simulink library "thc"  (R2021b)
settings: Solver=VariableStepAuto  StartTime=0.0  StopTime=10.0  RelTol=1e-3
undefined symbols (not defined in the file or in its folder): ATHC_APTCQA_X_C, ATHC_APTCQB_X_C, ATHC_dAy_X_C, ATHC_Qeq_X_kmh, ATHC_VbaseC_X_C, ATHC_VbaseC_Y_W, ATHC_VbaseD_X_C, ATHC_VbaseH_X_C, FALSE, KTHC_ACMaxMinT_sec, KTHC_aDeice_K, KTHC_AGSDefLv_K, KTHC_AGSLv1_K, KTHC_AGSLv2_K, KTHC_AGSLv3_K, KTHC_AGSLv4_K, KTHC_AGSLv5_K, KTHC_AirIntUpdateT_sec, KTHC_APTCOneZoneMax_W, KTHC_APTCPeriod_cnt, KTHC_APTCPWMEN_flg, KTHC_APTCQMaxC_W, KTHC_APTCQminC_W, KTHC_APTCQminD_W, KTHC_APTCQminRe1_W, KTHC_APTCQminRe_W, KTHC_APTCQoffT_cnt, KTHC_APTCQonT_cnt, KTHC_APTCRiLeMaxDff_W, KTHC_APTCRiLeMinDff_W, KTHC_BatInTempDef_C, KTHC_bDeice_K, KTHC_CompMaxDeice_rpm, KTHC_CompMinDeice_rpm, KTHC_CompSotxvOp_K, KTHC_CompSotxvOpLow_rpm, KTHC_CompSpdmax_rpm, KTHC_CompSpdmaxBC1_rpm, KTHC_CompSpdmaxBC_rpm, KTHC_CompSpdmid1_rpm, KTHC_CompSpdmid2_rpm, KTHC_CompSpdmid3_rpm, KTHC_CompSpdmid_rpm, KTHC_CompSpdmin_rpm, KTHC_DAPTCQ1_W, KTHC_DAPTCQ2_W, KTHC_DAPTCQ3_W, KTHC_DcChSetTemp_C, KTHC_DehumidityEN_flg, KTHC_DeiceCycTime_K, KTHC_DriveLevelWPTCBAH1_W, KTHC_DriveLevelWPTCBAH2_W, KTHC_DriveLevelWPTCBAH3_W, KTHC_DriveLevelWPTCBAH4_W, KTHC_DriveT1MinBAH_C, KTHC_DriveT2MaxBAH_C, KTHC_DriveT2MinBAH_C, KTHC_DriveT3MaxBAH_C, KTHC_DriveT3MinBAH_C, KTHC_DriveT4MaxBAH_C ... (+377)
libraries: simulink x145
(part 3 of 10)

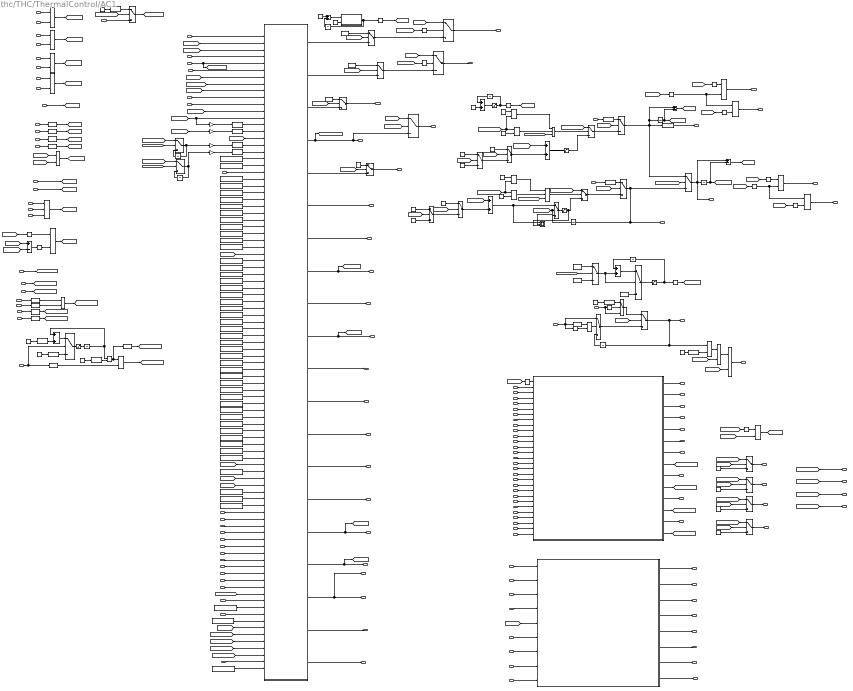
== system thc/THC/ThermalControl/AC1 ==
  VINP_FCPFrEvtBtnACMaxReq_flg : Inport
  VINP_FCPFrEvtBtnACReq_flg : Inport  Port=2
  VINP_FCPFrEvtBtnAutoReq_flg : Inport  Port=3
  VINP_FCPFrEvtBtnSyncReq_flg : Inport  Port=4
  VINP_Tamb_C : Inport  Port=5
  VINP_Tincar_C : Inport  Port=6
  VINP_sigAirIntenZon1Req_enum : Inport  Port=7
  VINP_sigRecircReq_flg : Inport  Port=8
  VINP_sigFaceReq_flg : Inport  Port=9
  VINP_sigFootReq_flg : Inport  Port=10
  VINP_sigFrostReq_flg : Inport  Port=11
  VINP_sigSetTempZon1Req_C : Inport  Port=12
  VINP_CANMsgValidIVI2_flg : Inport  Port=13
  VINP_sigSetTempZon2Req_C : Inport  Port=14
  VTHC_FDBlowerCmd_pct : Inport  Port=15
  PwrSta : Inport  Port=16
  OFF_AC_MODE : Inport  Port=17
  CabinMode : Inport  Port=18
  T_Foot_L : Inport  Port=19
  T_Foot_R : Inport  Port=20
  T_Foot_Rr : Inport  Port=21
  EEP_ACModeMem : Inport  Port=22
  EEP_Face : Inport  Port=23
  EEP_Foot : Inport  Port=24
  EEP_Frost : Inport  Port=25
  EEP_FaceM : Inport  Port=26
  EEP_FootM : Inport  Port=27
  EEP_CCUSyncSts : Inport  Port=28
  EEP_ACForceOFF : Inport  Port=29
  EEP_sigRecircSt : Inport  Port=30
  EEP_RecAutoFlg : Inport  Port=31
  EEP_AirIntenZone1M : Inport  Port=32
  EEP_fdefog : Inport  Port=33
  EEP_sigSetTempZon1Req : Inport  Port=34
  EEP_sigSetTempZon2StM : Inport  Port=35
  VINP_RemoteAutoReq_flg : Inport  Port=36
  ACSubMode : Inport  Port=37
  VINP_HMIACBtnCmd_flg : Inport  Port=38
  VINP_HMIACAutoBtnCmd_flg : Inport  Port=39
  VINP_HMIACRecycleBtnCmd_flg : Inport  Port=40
  VINP_HMIACFrDefogBtnCmd_flg : Inport  Port=41
  VINP_HMIZ1SetTPCmd_flg : Inport  Port=42
  VINP_HMIZ1SetTMCmd_flg : Inport  Port=43
  VINP_HMIZ2SetTPCmd_flg : Inport  Port=44
  VINP_HMIZ2SetTMCmd_flg : Inport  Port=45
  VINP_HMIACWindDirPCmd_flg : Inport  Port=46
  VINP_HMIACWindDirMCmd_flg : Inport  Port=47
  VINP_HMIACAirIntPCmd_flg : Inport  Port=48
  VINP_HMIACAirIntDirMCmd_flg : Inport  Port=49
  VINP_IVIAirIntZ3Cmd_enum : Inport  Port=50
  EEP_FDCTHCAirIntZ3Sta : Inport  Port=51
  VINP_IVIDrBlowerModeSta_enum : Inport  Port=52
  VINP_IVIPsBlowerModeSta_enum : Inport  Port=53
  VINP_IVIDrBlowerZSta_enum : Inport  Port=54
  VINP_IVICLBlowerZSta_enum : Inport  Port=55
  VINP_IVIPsBlowerZSta_enum : Inport  Port=56
  VINP_IVICRBlowerZSta_enum : Inport  Port=57
  VINP_IVIDrBlowerYSta_enum : Inport  Port=58
  VINP_IVICLBlowerYSta_enum : Inport  Port=59
  VINP_IVIPsBlowerYSta_enum : Inport  Port=60
  VINP_IVICRBlowerYSta_enum : Inport  Port=61
  VINP_ZFRTHCDrEVentActYSta_enum : Inport  Port=62
  VINP_ZFRTHCCLEVentActYSta_enum : Inport  Port=63
  VINP_ZFRTHCPsEVentActYSta_enum : Inport  Port=64
  VINP_ZFRTHCCREVentActYSta_enum : Inport  Port=65
  VINP_FDCTHCDrEVentModeStaM_enum : Inport  Port=66
  VINP_FDCTHCPsEVentModeStaM_enum : Inport  Port=67
  VINP_FDCTHCDrEVentZStaM_enum : Inport  Port=68
  VINP_FDCTHCCLEVentZStaM_enum : Inport  Port=69
  VINP_FDCTHCPsEVentZStaM_enum : Inport  Port=70
  VINP_FDCTHCCREVentZStaM_enum : Inport  Port=71
  EEP_DrVentENM : Inport  Port=72
  VINP_FDCTHCDrEVentYStaM_enum : Inport  Port=73
  EEP_CLVentENM : Inport  Port=74
  VINP_FDCTHCCLEVentYStaM_enum : Inport  Port=75
  EEP_PsVentENM : Inport  Port=76
  VINP_FDCTHCPsEVentYStaM_enum : Inport  Port=77
  EEP_CRVentENM : Inport  Port=78
  VINP_FDCTHCCREVentYStaM_enum : Inport  Port=79
  VINP_IVIsigScreenReq_Sta : Inport  Port=80
  VINP_IVIFGSAirIntCmd_enum : Inport  Port=81
  FGSAirIntStaM : Inport  Port=82
  VINP_IVIFGSChCmd_enum : Inport  Port=83
  FGSChStaM : Inport  Port=84
  VINP_IVIIONSWCmd_flg : Inport  Port=85
  "IONSWStaM " : Inport  Port=86
  VINP_FGSMotorInitSta_enum : Inport  Port=87
  VINP_FGSAirIntSta_enum : Inport  Port=88
  VINP_IVIZon1WindDirSWReqSta_flg : Inport  Port=89
  Add{,1..2,4..6} (6 alike) : Sum
  Add3 : Sum  Inputs=+-
  Add7 : Sum  Inputs=+-
  Add8 : Sum  Inputs=+-
  Chart : Stateflow chart  TreatAsAtomicUnit=on
      settings: PortSchema="{\"entries\":[{\"content\":{\"sides\":[{\"content\":{\"connectorIds\":[\"In1\",\"In2\",\"In3\",\"In4\",\"In5\",\"In6\",\"In7\",\"In8\",\"In9\",\"In10\",\"In11\",\"In12\",\"In13\",\"In14\",\"In15\",\"In16\",\"In18\",\"In17\",\"In19\",\"In20\",\"In21\",\"In22\",\"In23\",\"In24\",\"In25\",\"In26\",\"In27\",\"In28\",\"In29\",\"In30\",\"In31\",\"In32\",\"In33\",\"In34\",\"In35\",\"In36\",\"In37\",\"In38\",\"In39\",\"In40\",\"In41\",\"In42\",\"In43\",\"In44\",\"In45\",\"In46\",\"In47\",\"In48\",\"In49\",\"In50\",\"In51\",\"In52\",\"In53\",\"In54\",\"In55\",\"In56\",\"In57\",\"In58\",\"In59\",\"In60\",\"In61\",\"In62\",\"In63\",\"In64\",\"In65\",\"In66\",\"In67\",\"In68\",\"In69\",\"In70\",\"In71\",\"In72\",\"In73\",\"In74\",\"In75\",\"In76\",\"In77\",\"In78\",\"In79\",\"In80\",\"In81\",\"In82\",\"In83\",\"In84\",\"In85\",\"In86\",\"In87\",\"In88\",\"In89\",\"In90\",\"In91\",\"In92\",\"In93\",\"In94\"]},\"type\":\"ConnectorPlacement.EquallySpacedRectSide\",\"uuid\":\"5820fc40-35f0-4b43-a348-a95be02a5108\"},{\"content\":{\"connectorIds\":[\"Out1\",\"Out6\",\"Out2\",\"Out3\",\"Out4\",\"Out5\",\"Out7\",\"Out8\",\"Out9\",\"Out10\",\"Out11\",\"Out12\",\"Out13\",\"Out14\",\"Out15\",\"Out16\",\"Out17\",\"Out18\",\"Out19\",\"Out20\"],\"side\":\"RIGHT\"},\"type\":\"ConnectorPlacement.EquallySpacedRectSide\",\"uuid\":\"36d6613c-bf09-4a00-b7cd-6c94d14300cf\"},{\"content\":{\"connectorIds\":[],\"side\":\"TOP\"},\"type\":\"ConnectorPlacement.EquallySpacedRectSide\",\"uuid\":\"1ae2c247-46e8-45cc-9ea1-ac445f4d9fda\"}]},\"type\":\"ConnectorPlacement.EquallySpacedConnector\",\"uuid\":\"a8684177-dc23-416a-a392-32f98192c4b4\"}],\"packageUris\":[\"http://schema.mathworks.com/mf0/Connector/R2020b\"],\"version\":\"1.0\"}"
  Compare To Constant : simulink/Logic and Bit Operations/Compare To Constant  relop=<  const=5  OutDataTypeStr=boolean
  Compare To Constant1 : simulink/Logic and Bit Operations/Compare To Constant  relop=>=  const=1  OutDataTypeStr=boolean
  Compare To Constant10 : simulink/Logic and Bit Operations/Compare To Constant  relop=>  const=0  OutDataTypeStr=boolean
  Compare To Constant11 : simulink/Logic and Bit Operations/Compare To Constant  relop=<  const=0  OutDataTypeStr=boolean
  Compare To Constant12 : simulink/Logic and Bit Operations/Compare To Constant  relop=>  const=0  OutDataTypeStr=boolean
  Compare To Constant13 : simulink/Logic and Bit Operations/Compare To Constant  relop=<  const=0  OutDataTypeStr=boolean
  Compare To Constant2 : simulink/Logic and Bit Operations/Compare To Constant  relop=>=  const=100  OutDataTypeStr=boolean
  Compare To Constant3 : simulink/Logic and Bit Operations/Compare To Constant  relop===  const=3.0  OutDataTypeStr=boolean
  Compare To Constant4 : simulink/Logic and Bit Operations/Compare To Constant  relop=<  const=0  OutDataTypeStr=boolean
  Compare To Constant5 : simulink/Logic and Bit Operations/Compare To Constant  relop=<  const=3.0  OutDataTypeStr=boolean
  Compare To Constant6 : simulink/Logic and Bit Operations/Compare To Constant  relop===  const=2  OutDataTypeStr=boolean
  Compare To Constant7 : simulink/Logic and Bit Operations/Compare To Constant  relop===  const=1  OutDataTypeStr=boolean
  Compare To Constant8 : simulink/Logic and Bit Operations/Compare To Constant  relop===  const=0  OutDataTypeStr=boolean
  Compare To Constant9 : simulink/Logic and Bit Operations/Compare To Constant  relop=>  const=0  OutDataTypeStr=boolean
  Constant{,8,55,68,70..71} (6 alike) : Constant
  Constant1 : Constant  Value=10
  Constant10 : Constant  Value=KTHC_T2Mmaxamb_C
  Constant11 : Constant  Value=KTHC_T3Mmaxamb_C
  Constant12 : Constant  Value=KTHC_T4Mmaxamb_C
  Constant13 : Constant  Value=KTHC_T3Mminamb_C
  Constant14 : Constant  Value=KTHC_T4Mminamb_C
  Constant15 : Constant  Value=KTHC_T5Mminamb_C
  Constant16 : Constant  Value=KTHC_RecyHold_min
  Constant17 : Constant  Value=KTHC_RecyChange_min
  Constant18 : Constant  Value=KTHC_Tmidlevel_C
  Constant19 : Constant  Value=KTHC_Thilevel1_C
  Constant2 : Constant  Value=FALSE
  Constant20 : Constant  Value=KTHC_Thilevel2_C
  Constant21 : Constant  Value=KTHC_WDZ1Face_flg
  Constant22 : Constant  Value=KTHC_WDZ1Foot_flg
  Constant23 : Constant  Value=KTHC_WDZ1Frost_flg
  Constant24 : Constant  Value=KTHC_WDZ2Face_flg
  Constant25 : Constant  Value=KTHC_WDZ2Foot_flg
  Constant26 : Constant  Value=KTHC_WDZ2Frost_flg
  Constant27 : Constant  Value=KTHC_WDZ3Face_flg
  Constant28 : Constant  Value=KTHC_WDZ3Foot_flg
  Constant29 : Constant  Value=KTHC_WDZ3Frost_flg
  Constant3 : Constant  Value=FALSE
  Constant30 : Constant  Value=KTHC_WDZ4Face_flg
  Constant31 : Constant  Value=KTHC_WDZ4Foot_flg
  Constant32 : Constant  Value=KTHC_WDZ4Frost_flg
  Constant33 : Constant  Value=KTHC_WDZ5Face_flg
  Constant34 : Constant  Value=KTHC_WDZ5Foot_flg
  Constant35 : Constant  Value=KTHC_WDZ5Frost_flg
  Constant36 : Constant  Value=KTHC_WDZ6Face_flg
  Constant37 : Constant  Value=KTHC_WDZ6Foot_flg
  Constant38 : Constant  Value=KTHC_WDZ6Frost_flg
  Constant39 : Constant  Value=KTHC_WDZ7Face_flg
  Constant4 : Constant  Value=ZERO_INT
  Constant40 : Constant  Value=KTHC_WDZ7Foot_flg
  Constant41 : Constant  Value=KTHC_WDZ7Frost_flg
  Constant42 : Constant  Value=KTHC_WDZ8Face_flg
  Constant43 : Constant  Value=KTHC_WDZ8Foot_flg
  Constant44 : Constant  Value=KTHC_WDZ8Frost_flg
  Constant45 : Constant  Value=KTHC_WDZ9Face_flg
  Constant46 : Constant  Value=KTHC_WDZ9Foot_flg
  Constant47 : Constant  Value=KTHC_WDZ9Frost_flg
  Constant48 : Constant  Value=ONE_INT
  Constant49 : Constant  Value=ZERO_INT
  Constant5 : Constant  Value=KTHC_RecyOutterD_enum
  Constant50 : Constant  Value=KTHC_Trecymin_C
  Constant51 : Constant  Value=KTHC_RefreshEN_flg
  Constant52 : Constant  Value=KTHC_FootColdT_C
  Constant53 : Constant  Value=KTHC_FootColdTdelta_C
  Constant54 : Constant  Value=KTHC_ACMaxMinT_sec
  Constant56 : Constant  Value=FALSE
  Constant57 : Constant  Value=KTHC_WDZ10Foot_flg
  Constant58 : Constant  Value=KTHC_WDZ10Frost_flg
  Constant59 : Constant  Value=0.5
  Constant6 : Constant  Value=KTHC_WDZ10Face_flg
  Constant60 : Constant  Value=-0.5
  Constant61 : Constant  Value=0
  Constant62 : Constant  Value=0.5
  Constant63 : Constant  Value=-0.5
  Constant64 : Constant  Value=0
  Constant65 : Constant  Value=32
  Constant66 : Constant  Value=32
  Constant67 : Constant  Value=0
  Constant69 : Constant  Value=11
  Constant7 : Constant  Value=KTHC_WindDirUpdateT_min
  Constant{72..75} (4 alike) : Constant  Value=false
  Constant76 : Constant  Value=4
  Constant77 : Constant  Value=17
  Constant78 : Constant  Value=17
  Constant79 : Constant  Value=KTHC_ScreenUniq_flg
  Constant9 : Constant  Value=KTHC_AirIntUpdateT_sec
  Data Type Conversion : DataTypeConversion  OutDataTypeStr=single
  Data Type Conversion1 : DataTypeConversion  OutDataTypeStr=single
  Data Type Conversion{6..11} (6 alike) : DataTypeConversion  OutDataTypeStr=uint8
  Data Type Conversion12 : DataTypeConversion  OutDataTypeStr=single
  Data Type Conversion{2..5} (4 alike) : DataTypeConversion  OutDataTypeStr=uint16
  Detect Change : simulink/Logic and Bit Operations/Detect Change  vinit=0  OutDataTypeStr=boolean
  Detect Decrease : simulink/Logic and Bit Operations/Detect Decrease  vinit=0.0  OutDataTypeStr=boolean
  Detect Decrease1 : simulink/Logic and Bit Operations/Detect Decrease  vinit=0.0  OutDataTypeStr=boolean
  Detect Increase{,1..7} (8 alike) : simulink/Logic and Bit Operations/Detect Increase  vinit=0.0  OutDataTypeStr=boolean
  EVent : Subsystem
  Gain{,1..3} (4 alike) : Gain  Gain=10
  Logical Operator : Logic  Operator=NXOR  AllPortsSameDT=off  OutDataTypeStr=boolean
  Logical Operator{1..2,4..6,11,20} (7 alike) : Logic  Operator=OR  AllPortsSameDT=off  OutDataTypeStr=boolean
  Logical Operator{3,9..10,12..16} (8 alike) : Logic  AllPortsSameDT=off  OutDataTypeStr=boolean
  Logical Operator17 : Logic  Operator=NOT  AllPortsSameDT=off  OutDataTypeStr=boolean
  Logical Operator18 : Logic  Operator=NOT  AllPortsSameDT=off  OutDataTypeStr=boolean
  Logical Operator19 : Logic  Operator=NOT  AllPortsSameDT=off  OutDataTypeStr=boolean
  Logical Operator7 : Logic  Inputs=3  AllPortsSameDT=off  OutDataTypeStr=boolean
  Logical Operator8 : Logic  Inputs=3  AllPortsSameDT=off  OutDataTypeStr=boolean
  Min : MinMax  Inputs=3
  ModMath2 : Subsystem  mask(Count){}
      mask help: Counter function.
      mask Display:
      | fprintf('ModMath');
      | port_label('output', 1, 'Remainder');
      | port_label('input', 1, 'Dividend');
      | port_label('input', 2, 'Divisor');
  Relational Operator{,1,4..5} (4 alike) : RelationalOperator  Operator=<=  OutDataTypeStr=boolean  RndMeth=Simplest
  Relational Operator2 : RelationalOperator  Operator=<  OutDataTypeStr=boolean  RndMeth=Simplest
  Relational Operator3 : RelationalOperator  Operator=>  OutDataTypeStr=boolean  RndMeth=Simplest
  Saturation : Saturate  UpperLimit=100  LowerLimit=0
  Saturation1 : Saturate  UpperLimit=3  LowerLimit=0
  Saturation2 : Saturate  UpperLimit=32  LowerLimit=17
  Saturation3 : Saturate  UpperLimit=32  LowerLimit=17
  Saturation4 : Saturate  UpperLimit=12  LowerLimit=0
  Scope : Scope  NumInputPorts=3
  Subsystem : Subsystem
  Switch{,1..29} (30 alike) : Switch  Criteria=u2 > Threshold
  Unit Delay{,2,4..10} (9 alike) : UnitDelay  SampleTime=-1  HasFrameUpgradeWarning=on
  Unit Delay1 : UnitDelay  InitialCondition=26  SampleTime=-1  HasFrameUpgradeWarning=on
  VTHC_CCUACLampSts_flg : Outport
  VTHC_CCUAutoLampSts_flg : Outport  Port=2
  VTHC_CCUACMaxLampSts_flg : Outport  Port=3
  VTHC_CCUSyncLampSts_flg : Outport  Port=4
  VTHC_sigAirIntenZon1St_enum : Outport  Port=5
  VTHC_sigWindDirZon1St_enum : Outport  Port=6
  VTHC_sigRecircSt_flg : Outport  Port=7
  VTHC_sigSetTempZon1St_C : Outport  Port=8
  VTHC_sigSetTempZon2St_C : Outport  Port=9
  WaterFillReq : Outport  Port=10
  PET : Outport  Port=11
  FD_RecyAuto_Cmd : Outport  Port=12
  ACModeMem : Outport  Port=13
  Face : Outport  Port=14
  Foot : Outport  Port=15
  Frost : Outport  Port=16
  FaceM : Outport  Port=17
  FootM : Outport  Port=18
  CCUSyncSts : Outport  Port=19
  ACForceOFF : Outport  Port=20
  RecAutoFlg : Outport  Port=21
  AirIntenZone1M : Outport  Port=22
  fdefog : Outport  Port=23
  VTHC_sigSetTempZon2StM_C : Outport  Port=24
  VTHC_sigDfrstSt_flg : Outport  Port=25
  VTHC_FDCTHCAirIntZ3Sta_enum : Outport  Port=26
  RrAPTCEN : Outport  Port=27
  VTHC_FDCTHCDrEVentModeSta_enum : Outport  Port=28
  VTHC_FDCTHCPsEVentModeSta_enum : Outport  Port=29
  VTHC_FDCTHCDrEVentZSta_enum : Outport  Port=30
  VTHC_FDCTHCCLEVentZSta_enum : Outport  Port=31
  VTHC_FDCTHCPsEVentZSta_enum : Outport  Port=32
  VTHC_FDCTHCCREVentZSta_enum : Outport  Port=33
  VTHC_FDCTHCDrEVentYSta_enum : Outport  Port=34
  VTHC_FDCTHCDrVentENSta_flg : Outport  Port=35
  VTHC_FDCTHCCLEVentYSta_enum : Outport  Port=36
  VTHC_FDCTHCCLVentENSta_flg : Outport  Port=37
  VTHC_FDCTHCPsEVentYSta_enum : Outport  Port=38
  VTHC_FDCTHCPsVentENSta_flg : Outport  Port=39
  VTHC_FDCTHCCREVentYSta_enum : Outport  Port=40
  VTHC_FDCTHCCRVentENSta_flg : Outport  Port=41
  VTHC_DrVentEN_flg : Outport  Port=42
  VTHC_CLVentEN_flg : Outport  Port=43
  VTHC_PsVentEN_flg : Outport  Port=44
  VTHC_CRVentEN_flg : Outport  Port=45
  VTHC_Z1TUP_flg : Outport  Port=46
  VTHC_Z1TDN_flg : Outport  Port=47
  VTHC_Z2TUP_flg : Outport  Port=48
  VTHC_Z2TDN_flg : Outport  Port=49
  VTHC_FDCFGSAirIntSta_enum : Outport  Port=50
  VTHC_FDCFGSChSta_enum : Outport  Port=51
  VTHC_FDCFGSAirIntCmd_enum : Outport  Port=52
  VTHC_FDCFGSFuncSta_flg : Outport  Port=53
  VTHC_FDCFGSChCmd_enum : Outport  Port=54
  VTHC_FDCFGSIONSWSta_flg : Outport  Port=55
  VTHC_FDCFGSIONCmd_flg : Outport  Port=56
  VTHC_FDCFGSLearnCmd_enum : Outport  Port=57
  wires:
  Logical Operator16/1 -> VTHC_Z2TDN_flg/1  "VTHC_Z2TDN_flg"
  [Z2TempG] -> Compare To Constant13/1
  Logical Operator15/1 -> VTHC_Z2TUP_flg/1  "VTHC_Z2TUP_flg"
  Compare To Constant13/1 -> Logical Operator16/2
  Switch12/1 -> Unit Delay1/1, VTHC_sigSetTempZon2StM_C/1, Switch/3  "VTHC_sigSetTempZon2StM_C"
  Compare To Constant12/1 -> Logical Operator15/1
  [Z2TempG] -> Compare To Constant12/1
  Add8/1 -> [Z2TempG]
  Logical Operator19/1 -> Logical Operator16/1, Logical Operator15/2
  Logical Operator14/1 -> VTHC_Z1TDN_flg/1  "VTHC_Z1TDN_flg"
  [Z1TempG] -> Compare To Constant11/1
  Unit Delay10/1 -> [sigSetTempZon1St], Add7/2
  Switch11/1 -> Unit Delay10/1, Add7/1, Switch/1, Data Type Conversion12/1  "VTHC_sigSetTempZon1St_C"
  Add7/1 -> [Z1TempG]
  Compare To Constant11/1 -> Logical Operator14/2
  Compare To Constant10/1 -> Logical Operator13/1
  Logical Operator13/1 -> VTHC_Z1TUP_flg/1  "VTHC_Z1TUP_flg"
  Logical Operator17/1 -> Logical Operator14/1, Logical Operator13/2
  [Z1TempG] -> Compare To Constant10/1
  [DrVentEN] -> VTHC_DrVentEN_flg/1
  [CLVentEN] -> VTHC_CLVentEN_flg/1
  [PSVentEN] -> VTHC_PsVentEN_flg/1
  [CRVentEN] -> VTHC_CRVentEN_flg/1
  Data Type Conversion12/1 -> VTHC_sigSetTempZon1St_C/1  "VTHC_sigSetTempZon1St_C"
  VINP_IVIsigScreenReq_Sta/1 -> Chart/93(sigScreenReq)
  Logical Operator12/1 -> [EVACEN]
  [Face] -> Logical Operator12/2
  Compare To Constant9/1 -> Logical Operator12/1
  [VTHC_FDBlowerCmd_pct] -> Compare To Constant9/1
  Constant76/1 -> Data Type Conversion11/1
  Data Type Conversion11/1 -> Switch29/1
  EEP_FDCTHCAirIntZ3Sta/1 -> Compare To Constant8/1, Switch29/3
  Compare To Constant8/1 -> Switch29/2
  EVent/14(VTHC_FDCTHCCRVentEN_flg) -> [CRVentEN]
  [CRVentEN] -> Switch28/1
  [EVACEN] -> Switch28/2
  Constant75/1 -> Switch28/3
  EVent/12(VTHC_FDCTHCPsVentEN_flg) -> [PSVentEN]
  Constant74/1 -> Switch27/3
  [EVACEN] -> Switch27/2
  [PSVentEN] -> Switch27/1
  EVent/10(VTHC_FDCTHCCLVentEN_flg) -> [CLVentEN]
  [CLVentEN] -> Switch26/1
  [EVACEN] -> Switch26/2
  Constant73/1 -> Switch26/3
  Constant72/1 -> Switch25/3
  [EVACEN] -> Switch25/2
  [DrVentEN] -> Switch25/1
  EVent/8(VTHC_FDCTHCDrVentEN_flg) -> [DrVentEN]
  Switch25/1 -> VTHC_FDCTHCDrVentENSta_flg/1
  Switch28/1 -> VTHC_FDCTHCCRVentENSta_flg/1
  EVent/13(VTHC_FDCTHCCREVentYSta_enum) -> VTHC_FDCTHCCREVentYSta_enum/1
  Switch27/1 -> VTHC_FDCTHCPsVentENSta_flg/1
  EVent/11(VTHC_FDCTHCPsEVentYSta_enum) -> VTHC_FDCTHCPsEVentYSta_enum/1
  Switch26/1 -> VTHC_FDCTHCCLVentENSta_flg/1
  EVent/9(VTHC_FDCTHCCLEVentYSta_enum) -> VTHC_FDCTHCCLEVentYSta_enum/1
  EVent/7(VTHC_FDCTHCDrEVentYSta_enum) -> VTHC_FDCTHCDrEVentYSta_enum/1
  EVent/6(VTHC_FDCTHCCREVentZSta_enum) -> VTHC_FDCTHCCREVentZSta_enum/1
  EVent/5(VTHC_FDCTHCPsEVentZSta_enum) -> VTHC_FDCTHCPsEVentZSta_enum/1
  EVent/4(VTHC_FDCTHCCLEVentZSta_enum) -> VTHC_FDCTHCCLEVentZSta_enum/1
  EVent/3(VTHC_FDCTHCDrEVentZSta_enum) -> VTHC_FDCTHCDrEVentZSta_enum/1
  EVent/2(VTHC_FDCTHCPsEVentModeSta_enum) -> VTHC_FDCTHCPsEVentModeSta_enum/1
  EVent/1(VTHC_FDCTHCDrEVentModeSta_enum) -> VTHC_FDCTHCDrEVentModeSta_enum/1
  Logical Operator11/1 -> RrAPTCEN/1
  [Foot] -> Logical Operator11/2
  Logical Operator10/1 -> Logical Operator11/1
  Relational Operator3/1 -> Logical Operator10/1
  [Face] -> Logical Operator10/2
  Data Type Conversion10/1 -> Relational Operator3/2
  Constant71/1 -> Data Type Conversion10/1
  VINP_FDCTHCCREVentYStaM_enum/1 -> EVent/29(VINP_FDCTHCCREVentYStaM_enum)
  EEP_CRVentENM/1 -> EVent/28(VTHC_FDCTHCCRVentENM_flg)
  VINP_FDCTHCPsEVentYStaM_enum/1 -> EVent/26(VINP_FDCTHCPsEVentYStaM_enum)
  EEP_PsVentENM/1 -> EVent/25(VTHC_FDCTHCPsVentENM_flg)
  VINP_FDCTHCCLEVentYStaM_enum/1 -> EVent/21(VINP_FDCTHCCLEVentYStaM_enum)
  EEP_CLVentENM/1 -> EVent/20(VTHC_FDCTHCCLVentENM_flg)
  VINP_FDCTHCDrEVentYStaM_enum/1 -> EVent/18(VINP_FDCTHCDrEVentYStaM_enum)
  EEP_DrVentENM/1 -> EVent/17(VTHC_FDCTHCDrVentENM_flg)
  VINP_FDCTHCCREVentZStaM_enum/1 -> EVent/13(VINP_FDCTHCCREVentZStaM_enum)
  VINP_FDCTHCPsEVentZStaM_enum/1 -> EVent/12(VINP_FDCTHCPsEVentZStaM_enum)
  VINP_FDCTHCCLEVentZStaM_enum/1 -> EVent/11(VINP_FDCTHCCLEVentZStaM_enum)
  VINP_FDCTHCDrEVentZStaM_enum/1 -> EVent/10(VINP_FDCTHCDrEVentZStaM_enum)
  VINP_FDCTHCPsEVentModeStaM_enum/1 -> EVent/5(VINP_FDCTHCPsEVentModeStaM_enum)
  VINP_FDCTHCDrEVentModeStaM_enum/1 -> EVent/3(VINP_FDCTHCDrEVentModeStaM_enum)
  VINP_ZFRTHCCREVentActYSta_enum/1 -> EVent/27(VINP_ZFRTHCCREVentActYSta_enum)
  VINP_ZFRTHCPsEVentActYSta_enum/1 -> EVent/24(VINP_ZFRTHCPsEVentActYSta_enum)
  VINP_ZFRTHCCLEVentActYSta_enum/1 -> EVent/19(VINP_ZFRTHCCLEVentActYSta_enum)
  VINP_ZFRTHCDrEVentActYSta_enum/1 -> EVent/16(VINP_ZFRTHCDrEVentActYSta_enum)
  VINP_IVICRBlowerYSta_enum/1 -> EVent/23(VINP_IVICRBlowerYSta_enum)
  VINP_IVIPsBlowerYSta_enum/1 -> EVent/22(VINP_IVIPsBlowerYSta_enum)
  VINP_IVICLBlowerYSta_enum/1 -> EVent/15(VINP_IVICLBlowerYSta_enum)
  VINP_IVIDrBlowerYSta_enum/1 -> EVent/14(VINP_IVIDrBlowerYSta_enum)
  VINP_IVICRBlowerZSta_enum/1 -> EVent/9(VINP_IVICRBlowerZSta_enum)
  VINP_IVIPsBlowerZSta_enum/1 -> EVent/8(VINP_IVIPsBlowerZSta_enum)
  VINP_IVICLBlowerZSta_enum/1 -> EVent/7(VINP_IVICLBlowerZSta_enum)
  VINP_IVIDrBlowerZSta_enum/1 -> EVent/6(VINP_IVIDrBlowerZSta_enum)
  VINP_IVIPsBlowerModeSta_enum/1 -> EVent/4(VINP_IVIPsBlowerModeSta_enum)
  VINP_IVIDrBlowerModeSta_enum/1 -> EVent/2(VINP_IVIDrBlowerModeSta_enum)
  [fInitial] -> Logical Operator18/1
  Switch24/1 -> VTHC_FDCTHCAirIntZ3Sta_enum/1, Relational Operator3/1, Unit Delay9/1  "VTHC_FDCTHCAirIntZ3Sta_enum"
  Switch23/1 -> Switch24/3
  [fInitial] -> Switch24/2
  Switch29/1 -> Switch24/1
  Unit Delay9/1 -> Switch23/3
  Compare To Constant1/1 -> Logical Operator3/2
  Logical Operator3/1 -> Switch23/2
  Detect Change/1 -> Logical Operator3/1
  VINP_IVIAirIntZ3Cmd_enum/1 -> Detect Change/1, Compare To Constant1/1, Switch23/1
  [sigAirIntenZon1Req] -> Chart/8(sigAirIntenZon1Req)
  Switch22/1 -> [sigAirIntenZon1Req]
  Constant70/1 -> Data Type Conversion9/1
  Data Type Conversion9/1 -> Switch22/1
  [AirIntOFF] -> Switch22/2
  Detect Decrease1/1 -> [AirIntOFF]
  Data Type Conversion8/1 -> Relational Operator2/2
  Constant69/1 -> Data Type Conversion8/1
  Relational Operator2/1 -> Logical Operator9/1, Detect Decrease1/1
  Logical Operator9/1 -> [AirIntM]
  Unit Delay/1 -> Relational Operator2/1, Add6/1
  Saturation4/1 -> Unit Delay/1
  Switch21/1 -> Saturation4/1
  Data Type Conversion7/1 -> Add6/2
  Constant68/1 -> Data Type Conversion7/1
  Add6/1 -> Switch21/1
  Constant67/1 -> Data Type Conversion6/1
  Data Type Conversion6/1 -> Switch21/3
  [AirIntM] -> Chart/92(AirIntM)
  [AirIntP] -> Chart/91(AirIntP)
  [WindDirM] -> Chart/90(WindDirM)
  [WindDirP] -> Chart/89(WindDirP)
  Detect Decrease/1 -> Logical Operator9/2
  Detect Increase6/1 -> [AirIntP]
  Detect Increase5/1 -> [WindDirM]
  Detect Increase4/1 -> Logical Operator20/1
  VINP_HMIACAirIntPCmd_flg/1 -> Detect Increase6/1
  VINP_HMIACAirIntDirMCmd_flg/1 -> Detect Decrease/1, Switch21/2
  VINP_HMIACWindDirMCmd_flg/1 -> Detect Increase5/1
  VINP_HMIACWindDirPCmd_flg/1 -> Detect Increase4/1
  [VINP_sigSetTempZon2Req_C] -> Relational Operator4/2, Relational Operator1/1
  Constant66/1 -> Relational Operator1/2
  Relational Operator1/1 -> Logical Operator8/2
  [VINP_CANMsgValidIVI2_flg] -> Logical Operator8/3
  Logical Operator8/1 -> Switch2/2
  [VINP_sigSetTempZon2Req_C] -> Switch2/1
  [VINP_sigSetTempZon1Req_C] -> Switch1/1
  Constant65/1 -> Relational Operator/2
  Relational Operator/1 -> Logical Operator7/2
  Logical Operator7/1 -> Switch1/2
  Saturation3/1 -> Scope/3, Switch2/3
  Saturation2/1 -> Switch1/3
  Switch20/1 -> Saturation3/1
  [SyncCancel] -> Scope/2, Switch20/2
  Add5/1 -> Scope/1, Switch20/1
  Unit Delay1/1 -> Switch20/3
  [sigSetTempZon2St] -> Add5/1
  [Z2SetTP] -> Switch18/2
  Constant62/1 -> Switch18/1
  Switch19/1 -> Switch18/3
  Switch18/1 -> Add5/2
  [Z2SetTM] -> Switch19/2
  Constant63/1 -> Switch19/1
  Constant64/1 -> Switch19/3
  Constant61/1 -> Switch17/3
  Constant60/1 -> Switch17/1
  [Z1SetTM] -> Switch17/2
  Switch16/1 -> Add1/2
  Switch17/1 -> Switch16/3
  Constant59/1 -> Switch16/1
  [Z1SetTP] -> Switch16/2
  Add1/1 -> Saturation2/1
  [sigSetTempZon1St] -> Add1/1
  [VINP_CANMsgValidIVI2_flg] -> Switch9/2
  [VINP_CANMsgValidIVI2_flg] -> Logical Operator7/3
  [SyncCancel] -> Chart/88(SyncCancel)
  Logical Operator6/1 -> [SyncCancel]
  [Z2SetTM] -> Logical Operator6/2
  [Z2SetTP] -> Logical Operator6/1
  VINP_HMIZ2SetTPCmd_flg/1 -> Detect Increase2/1
  Detect Increase2/1 -> [Z2SetTP]
  Detect Increase3/1 -> [Z2SetTM]
  VINP_HMIZ2SetTMCmd_flg/1 -> Detect Increase3/1
  VINP_HMIZ1SetTMCmd_flg/1 -> Detect Increase1/1
  Detect Increase1/1 -> [Z1SetTM]
  Detect Increase/1 -> [Z1SetTP]
  VINP_HMIZ1SetTPCmd_flg/1 -> Detect Increase/1
  [FrDefogBtn] -> Chart/12(sigFrostReq)
  Logical Operator5/1 -> [FrDefogBtn]
  VINP_sigFrostReq_flg/1 -> Logical Operator5/1
  VINP_HMIACFrDefogBtnCmd_flg/1 -> Logical Operator5/2
  [RecycleBtn] -> Chart/9(sigRecircReq)
  Logical Operator4/1 -> [RecycleBtn]
  VINP_sigRecircReq_flg/1 -> Logical Operator4/1
  VINP_HMIACRecycleBtnCmd_flg/1 -> Logical Operator4/2
  VINP_FCPFrEvtBtnSyncReq_flg/1 -> Chart/4(FCP_FrEvt_BtnSyncReq)
  [ACAUTOBtn] -> Chart/3(FCP_FrEvt_BtnAutoReq)
  Logical Operator2/1 -> [ACAUTOBtn]
  VINP_HMIACAutoBtnCmd_flg/1 -> Logical Operator2/2
  VINP_FCPFrEvtBtnAutoReq_flg/1 -> Logical Operator2/1
  [ACBtn] -> Chart/2(FCP_FrEvt_BtnACReq)
  Logical Operator1/1 -> [ACBtn]
  VINP_HMIACBtnCmd_flg/1 -> Logical Operator1/2
  VINP_FCPFrEvtBtnACReq_flg/1 -> Logical Operator1/1
  Constant58/1 -> Chart/63(KTHC_WDZ10Frost_flg)
  Constant57/1 -> Chart/62(KTHC_WDZ10Foot_flg)
  Constant6/1 -> Chart/61(KTHC_WDZ10Face_flg)
  [VINP_CANMsgValidIVI2_flg] -> Switch15/2
  [VINP_sigSetTempZon2Req_C] -> Switch15/1
  Unit Delay8/1 -> Switch15/3
  Switch15/1 -> Unit Delay8/1, Gain3/1
  [VINP_CANMsgValidIVI2_flg] -> Switch14/2
  Unit Delay5/1 -> Switch14/3
  [VINP_sigSetTempZon1Req_C] -> Switch14/1
  Constant5/1 -> Chart/87(KTHC_RecyOutterD_enum)
  Data Type Conversion5/1 -> Chart/17(sigSetTempZon2Req_CMD)
  Gain3/1 -> Data Type Conversion5/1
  Gain2/1 -> Data Type Conversion4/1
  Data Type Conversion4/1 -> Chart/18(sigSetTempZon1Req_CMD)
  Switch14/1 -> Gain2/1, Unit Delay5/1
  ACSubMode/1 -> Chart/86(ACSubMode)
  Constant50/1 -> Chart/85(KTHC_Trecymin_C)
  Compare To Constant7/1 -> Switch3/2
  Compare To Constant6/1 -> Switch13/2
  [WaterFillReq] -> Compare To Constant6/1
  Switch13/1 -> VTHC_CCUAutoLampSts_flg/1  "VTHC_CCUAutoLampSts_flg"
  [Flash] -> Switch13/1
  [Flash] -> Switch3/1
  Compare To Constant/1 -> [Flash]
  Switch6/1 -> Switch13/3  "VTHC_CCUAutoLampSts_flg"
  Chart/6(CCU_AutoLampSts) -> Switch6/3  "VTHC_CCUAutoLampSts_flg"
  VINP_RemoteAutoReq_flg/1 -> Chart/84(VINP_RemoteAutoReq_flg)
  Gain1/1 -> Data Type Conversion3/1
  [sigSetTempZon2St] -> Gain1/1
  Data Type Conversion3/1 -> Chart/15(SetTempZon2St_CMD)
  [sigSetTempZon1St] -> Gain/1, Chart/13(sigSetTempZon1St)
  Data Type Conversion2/1 -> Chart/14(SetTempZon1St_CMD)
  Gain/1 -> Data Type Conversion2/1
  Data Type Conversion1/1 -> Switch12/1
  Data Type Conversion/1 -> Switch11/1
  ModMath2/1(Remainder) -> Compare To Constant/1, Unit Delay4/1
  Unit Delay7/1 -> [sigSetTempZon2St], Add8/2
  [VINP_CANMsgValidIVI2_flg] -> Chart/83(VINP_CANMsgValidIVI2_flg)
  EEP_sigSetTempZon2StM/1 -> Data Type Conversion1/1
  [fInitial] -> Switch12/2
  Switch2/1 -> Switch12/3
  EEP_sigSetTempZon1Req/1 -> Data Type Conversion/1
  [fInitial] -> Switch11/2
  Switch1/1 -> Switch11/3
  Compare To Constant5/1 -> [fInitial]
  Unit Delay2/1 -> Add4/1
  Saturation1/1 -> Compare To Constant5/1, Unit Delay2/1
  Constant55/1 -> Add4/2
  Add4/1 -> Saturation1/1
  Chart/20(AirIntenZone1M) -> AirIntenZone1M/1
  Chart/19(RecAutoFlg) -> RecAutoFlg/1
  Chart/18(fdefog) -> VTHC_sigDfrstSt_flg/1, fdefog/1  "VTHC_sigDfrstSt_flg"
  EEP_fdefog/1 -> Chart/82(EEP_fdefog)
  Chart/17(Foot) -> Foot/1, [Foot]
  Chart/16(Face) -> Face/1, [Face]
  Chart/15(FootM) -> FootM/1
  Chart/14(FaceM) -> FaceM/1
  Chart/13(ACModeMem) -> ACModeMem/1
  EEP_AirIntenZone1M/1 -> Chart/81(EEP_AirIntenZone1M)
  EEP_RecAutoFlg/1 -> Chart/80(EEP_RecAutoFlg)
  EEP_sigRecircSt/1 -> Chart/79(EEP_sigRecircSt)
  EEP_ACForceOFF/1 -> Chart/78(EEP_ACForceOFF)
  EEP_CCUSyncSts/1 -> Chart/77(EEP_CCUSyncSts)
  EEP_FootM/1 -> Chart/76(EEP_FootM)
  EEP_FaceM/1 -> Chart/75(EEP_FaceM)
  EEP_Frost/1 -> Chart/74(EEP_Frost)
  EEP_Foot/1 -> Chart/73(EEP_Foot)
  EEP_Face/1 -> Chart/72(EEP_Face)
  EEP_ACModeMem/1 -> Chart/71(EEP_ACModeMem)
  Constant54/1 -> Chart/70(KTHC_ACMaxMinT_sec)
  [MaxFinish] -> Chart/66(MaxFinish)
  Logical Operator/1 -> [MaxFinish]
  Compare To Constant4/1 -> Logical Operator/2
  Compare To Constant3/1 -> Logical Operator/1
  Add3/1 -> Compare To Constant4/1
  [sigSetTempZon1St] -> Add3/2
  [Tincar] -> Add3/1
  [Tincar] -> Chart/7(Tincar)
  VINP_Tincar_C/1 -> [Tincar]
  [CabinMode] -> Compare To Constant3/1
  [CabinMode] -> Chart/33(CabinMode)
  CabinMode/1 -> [CabinMode]
  Constant53/1 -> Chart/69(KTHC_FootColdTdelta_C)
  Constant52/1 -> Chart/68(KTHC_FootColdT_C)
  [T_Foot_min] -> Chart/67(T_Foot_min)
  Min/1 -> [T_Foot_min]
  T_Foot_Rr/1 -> Min/3
  T_Foot_R/1 -> Min/2
  T_Foot_L/1 -> Min/1
  Constant51/1 -> Chart/65(KTHC_RefreshEN_flg)
  [ForceAuto] -> Chart/64(ForceAuto)
  Compare To Constant2/1 -> [ForceAuto]
  Saturation/1 -> Unit Delay6/1, Compare To Constant2/1
  Unit Delay6/1 -> Add2/1
  Switch10/1 -> Saturation/1
  Constant4/1 -> Switch10/3
  Add2/1 -> Switch10/1
  Switch9/1 -> Add2/2, Switch10/2
  Constant48/1 -> Switch9/3
  Constant49/1 -> Switch9/1
  Constant47/1 -> Chart/60(KTHC_WDZ9Frost_flg)
  Constant46/1 -> Chart/59(KTHC_WDZ9Foot_flg)
  Constant45/1 -> Chart/58(KTHC_WDZ9Face_flg)
  Constant44/1 -> Chart/57(KTHC_WDZ8Frost_flg)
  Constant43/1 -> Chart/56(KTHC_WDZ8Foot_flg)
  Constant42/1 -> Chart/55(KTHC_WDZ8Face_flg)
  Constant41/1 -> Chart/54(KTHC_WDZ7Frost_flg)
  Constant40/1 -> Chart/53(KTHC_WDZ7Foot_flg)
  Constant39/1 -> Chart/52(KTHC_WDZ7Face_flg)
  Constant38/1 -> Chart/51(KTHC_WDZ6Frost_flg)
  Constant37/1 -> Chart/50(KTHC_WDZ6Foot_flg)
  Constant36/1 -> Chart/49(KTHC_WDZ6Face_flg)
  Constant35/1 -> Chart/48(KTHC_WDZ5Frost_flg)
  Constant34/1 -> Chart/47(KTHC_WDZ5Foot_flg)
  Constant33/1 -> Chart/46(KTHC_WDZ5Face_flg)
  Constant32/1 -> Chart/45(KTHC_WDZ4Frost_flg)
  Constant31/1 -> Chart/44(KTHC_WDZ4Foot_flg)
  Constant30/1 -> Chart/43(KTHC_WDZ4Face_flg)
  Constant29/1 -> Chart/42(KTHC_WDZ3Frost_flg)
  Constant28/1 -> Chart/41(KTHC_WDZ3Foot_flg)
  Constant27/1 -> Chart/40(KTHC_WDZ3Face_flg)
  Constant26/1 -> Chart/39(KTHC_WDZ2Frost_flg)
  Constant25/1 -> Chart/38(KTHC_WDZ2Foot_flg)
  Constant24/1 -> Chart/37(KTHC_WDZ2Face_flg)
  Constant22/1 -> Chart/35(KTHC_WDZ1Foot_flg)
  Constant23/1 -> Chart/36(KTHC_WDZ1Frost_flg)
  Constant21/1 -> Chart/34(KTHC_WDZ1Face_flg)
  Constant20/1 -> Chart/32(KTHC_Thilevel2_C)
  Constant19/1 -> Chart/31(KTHC_Thilevel1_C)
  Constant18/1 -> Chart/30(KTHC_Tmidlevel_C)
  Chart/12(FD_RecyAuto_Cmd) -> FD_RecyAuto_Cmd/1
  Constant17/1 -> Chart/29(KTHC_RecyChange_min)
  Constant16/1 -> Chart/28(KTHC_RecyHold_min)
  Constant15/1 -> Chart/27(KTHC_T5Mminamb_C)
  Constant14/1 -> Chart/26(KTHC_T4Mminamb_C)
  Constant13/1 -> Chart/25(KTHC_T3Mminamb_C)
  Constant12/1 -> Chart/24(KTHC_T4Mmaxamb_C)
  Constant11/1 -> Chart/23(KTHC_T3Mmaxamb_C)
  Constant10/1 -> Chart/22(KTHC_T2Mmaxamb_C)
  Chart/11(PET) -> PET/1
  OFF_AC_MODE/1 -> Chart/21(OFF_AC_MODE)
  Constant9/1 -> Chart/20(KTHC_AirIntUpdateT_sec)
  VINP_sigSetTempZon1Req_C/1 -> [VINP_sigSetTempZon1Req_C]
  VINP_sigSetTempZon2Req_C/1 -> [VINP_sigSetTempZon2Req_C]
  Chart/4(sigAirIntenZon1St) -> Switch8/3
  Switch8/1 -> VTHC_sigAirIntenZon1St_enum/1  "VTHC_sigAirIntenZon1St_enum"
  [ACForceOFF] -> Switch8/2
  Constant8/1 -> Switch8/1
  Constant7/1 -> Chart/19(KTHC_WindDirUpdateT_min)
  Switch7/1 -> VTHC_CCUSyncLampSts_flg/1  "VTHC_CCUSyncLampSts_flg"
  [ACForceOFF] -> Switch7/2
  [Flash] -> Switch7/1
  Chart/3(CCU_SyncSts) -> CCUSyncSts/1, Switch7/3, [VTHC_CCUSyncSts_flg]
  Constant56/1 -> Switch6/1
  [ACForceOFF] -> Switch6/2
  Switch3/1 -> VTHC_CCUACLampSts_flg/1  "VTHC_CCUACLampSts_flg"
  Constant3/1 -> Switch5/1
  [ACForceOFF] -> Switch5/2
  Switch5/1 -> VTHC_CCUACMaxLampSts_flg/1  "VTHC_CCUACMaxLampSts_flg"
  Constant2/1 -> Switch4/1
  Switch4/1 -> Switch3/3  "VTHC_CCUACLampSts_flg"
  [ACForceOFF] -> Switch4/2
  Chart/10(ACForceOFF) -> ACForceOFF/1, [ACForceOFF]
  [WaterFillReq] -> Compare To Constant7/1
  Constant1/1 -> ModMath2/2(Divisor)
  Constant/1 -> Add/1
  Unit Delay4/1 -> Add/2
  Add/1 -> ModMath2/1(Dividend)
  Chart/8(WaterFillReq) -> WaterFillReq/1, [WaterFillReq]
  Chart/9(Frost) -> Frost/1
  VTHC_FDBlowerCmd_pct/1 -> Chart/5(FD_Blower_Cmd), [VTHC_FDBlowerCmd_pct]
  Chart/2(CCU_ACMaxLampSts) -> Switch5/3  "VTHC_CCUACMaxLampSts_flg"
  VINP_CANMsgValidIVI2_flg/1 -> [VINP_CANMsgValidIVI2_flg]  "VINP_CANMsgValidIVI2_flg"
  VINP_sigFootReq_flg/1 -> Chart/11(sigFootReq)
  VINP_sigFaceReq_flg/1 -> Chart/10(sigFaceReq)
  Switch/1 -> Add8/1, Unit Delay7/1, VTHC_sigSetTempZon2St_C/1  "VTHC_sigSetTempZon2St_C"
  Chart/5(sigWindDirZon1St) -> VTHC_sigWindDirZon1St_enum/1  "VTHC_sigWindDirZon1St_enum"
  VINP_FCPFrEvtBtnACMaxReq_flg/1 -> Chart/1(FCP_FrEvt_BtnACMaxReq)
  Chart/1(CCU_ACLampSts) -> Switch4/3  "VTHC_CCUACLampSts_flg"
  Chart/7(sigRecircSt) -> VTHC_sigRecircSt_flg/1  "VTHC_sigRecircSt_flg"
  VINP_sigAirIntenZon1Req_enum/1 -> Switch22/3
  VINP_Tamb_C/1 -> Chart/6(Tamb)
  [VTHC_CCUSyncSts_flg] -> Switch/2
  [fInitial] -> Logical Operator17/1
  [fInitial] -> Logical Operator19/1
  Constant77/1 -> Relational Operator4/1
  Relational Operator4/1 -> Logical Operator8/1
  Relational Operator5/1 -> Logical Operator7/1
  Constant78/1 -> Relational Operator5/1
  [VINP_sigSetTempZon1Req_C] -> Relational Operator5/2, Relational Operator/1
  VINP_IVIFGSAirIntCmd_enum/1 -> Subsystem/1(IVI_FGSAirInt_Cmd)
  FGSAirIntStaM/1 -> Subsystem/2(FGSAirIntStaM)
  VINP_IVIFGSChCmd_enum/1 -> Subsystem/3(IVI_FGSCh_Cmd)
  FGSChStaM/1 -> Subsystem/4(FGSChStaM)
  PwrSta/1 -> [PwrSta]
  [PwrSta] -> Chart/16(PwrSta)
  [PwrSta] -> Subsystem/5(PwrSta)
  VINP_IVIIONSWCmd_flg/1 -> Subsystem/6(IVI_IONSW_Cmd)
  "IONSWStaM "/1 -> Subsystem/7("IONSWStaM ")
  VINP_FGSMotorInitSta_enum/1 -> Subsystem/8(FGS_MotorInit_Sta)
  VINP_FGSAirIntSta_enum/1 -> Subsystem/9(FGS_AirInt_Sta)
  Subsystem/1(FGSAirIntSta) -> VTHC_FDCFGSAirIntSta_enum/1  "VTHC_FDCFGSAirIntSta_enum"
  Subsystem/2(FGSChSta) -> VTHC_FDCFGSChSta_enum/1  "VTHC_FDCFGSChSta_enum"
  Subsystem/3(FGSAirIntCmd) -> VTHC_FDCFGSAirIntCmd_enum/1  "VTHC_FDCFGSAirIntCmd_enum"
  Subsystem/4(FGSFuncSta) -> VTHC_FDCFGSFuncSta_flg/1  "VTHC_FDCFGSFuncSta_flg"
  Subsystem/5(FGSChCmd) -> VTHC_FDCFGSChCmd_enum/1  "VTHC_FDCFGSChCmd_enum"
  Subsystem/6(FDC_FGS_IONSW_Sta) -> VTHC_FDCFGSIONSWSta_flg/1  "VTHC_FDCFGSIONSWSta_flg"
  Subsystem/7(FDC_FGS_ION_Cmd) -> VTHC_FDCFGSIONCmd_flg/1  "VTHC_FDCFGSIONCmd_flg"
  Subsystem/8(FGSLearn) -> VTHC_FDCFGSLearnCmd_enum/1  "VTHC_FDCFGSLearnCmd_enum"
  Logical Operator18/1 -> EVent/1(fInitial)
  VINP_IVIZon1WindDirSWReqSta_flg/1 -> Detect Increase7/1
  Detect Increase7/1 -> Logical Operator20/2
  Logical Operator20/1 -> [WindDirP]
  Constant79/1 -> Chart/94(KTHC_ScreenUniq_flg)
